simulink library "commsink2"  (Simulink 6.0)
settings: Solver=ode45  SolverMode=SingleTasking  StartTime=0.0  StopTime=10.0  RelTol=1e-3
undefined symbols (not defined in the file or in its folder): commblkeyescat2, get, sdspfscope2
libraries: simulink x6, dspsigattribs x6, dspbuff3 x3, dspsnks4 x3, dspsrcs4 x3, dspsigops x3
settings Model: CovMetricSettings=d  Creator=tdelve  LastModifiedBy=mmclerno  ExtModeAutoUpdateStatusClock=off  UpdateModelReferenceTargets=IfOutOfDate
settings Model: ForwardingTableString=|
  | ||__slOldName__||commsink2/Continuous-Time
  | Eye and Scatter
  | Diagrams||__slNewName__||cbobsv2p5/Continuous-Time
  | Eye and Scatter
  | Diagrams||__slOldName__||commsink2/Triggered Write to File||__slNewName__||cbobsv2p5/Triggered Write to File||__slOldName__||commsink2/Error Rate Calculation||__slNewName__||commsink2/Error Rate
  | Calculation||__slOldName__||commsink2/Discrete-Time
  | Eye and Scatter
  | Diagrams||__slNewName__||cbobsv2/Discrete-Time
  | Eye and Scatter
  | Diagrams
settings DataIOCC: SignalLoggingName=logsOut
settings OptimizationCC: BooleanDataType=off
settings DebuggingCC: CheckExecutionContextPreStartOutputMsg=on  CheckExecutionContextRuntimeOutputMsg=on  SolverPrmCheckMsg=none
settings HardwareCC: TargetUnknown=on
settings ModelReferenceCC: UpdateModelReferenceTargets=IfOutOfDate
settings GRTTargetCC: UtilityFuncGeneration=Automatic  LifeSpan=inf
settings SFSimCC: SFSimApplyToAllLibs=on  SFSimBuildMode=Incremental

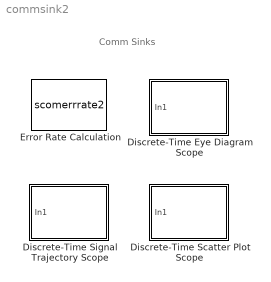
== system commsink2 ==
  note: Comm Sinks
  Discrete-Time Eye Diagram Scope : Subsystem  Tag=EyeDiagram  LoadFcn=commblkeyescat2(gcb,'Load');  StopFcn=sdspfscope2([],[],[],'StopBlock',[],[]);  EnableExecutionContextPropagation=on  mask(Discrete-Time Eye Diagram Scope){sampPerSymb=8, offsetEye=0, symbPerTrace=1, numTraces=40, numNewFrames=10, LineMarkers=, LineStyles=-, LineColors=b, dupPoints=on, fading=on, render=on, AxisGrid=on, yMin=-1.5, yMax=1.5, inphaseLabel=In-phase Amplitude, quadratureLabel=Quadrature Amplitude, openScopeAtSimStart=on, dispDiagram=In-phase and Quadrature, FrameNumber=off, FigPos=get(0,'defaultfigureposition');, figTitle=Eye Diagram, block_type_=eye, numLinesMax=8}
      mask prompts: sampPerSymb "Samples per symbol:"; offsetEye "Offset (samples):"; symbPerTrace "Symbols per trace:"; numTraces "Traces displayed:"; numNewFrames "New traces per display:"; LineMarkers "Markers:"; LineStyles "Line style:"; LineColors "Line color:"; dupPoints "Duplicate points at trace boundary"; fading "Color fading"; render "High quality rendering"; AxisGrid "Show grid"; yMin "Y axis minimum:"; yMax "Y axis maximum:"; inphaseLabel "In-phase Y-axis label:"; quadratureLabel "Quadrature Y-axis label:"; openScopeAtSimStart "Open scope at start of simulation"; dispDiagram "Eye diagram to display:"; FrameNumber "Trace number"; FigPos "Scope position:"; figTitle "Title:"; block_type_ "Block select"; numLinesMax "Max Num Lines"
      mask help:
      | The Discrete-Time Eye Diagram Scope displays multiple traces of a modulated signal to reveal the modulation characteristics such as pulse shaping, as well as channel distortions of the signal.
      |
      |
      | The signal is divided into traces with length, 'Samples per symbol'  * 'Symbols per trace' starting by skipping 'Offset' samples at the beginning.
      mask init:
      | commblkeyescat2(gcb,'init','eye');
      settings: OpenFcn=dspblkfscope2('dynamic','OpenScope');
      mask Help: helpview(commbhelp)
      mask StyleString: edit,edit,edit,edit,edit,edit,edit,edit,checkbox,checkbox,checkbox,checkbox,edit,edit,edit,edit,checkbox,popup(In-phase Only|In-phase and Quadrature),checkbox,edit,edit,popup(eye|scatter|xy),edit
      mask CallbackString: |||||||||||||||||commblkeyescat2(gcb,'cbDispDiagram');|||||
      mask TabNameString: Plotting Properties,Plotting Properties,Plotting Properties,Plotting Properties,Plotting Properties,Rendering Properties,Rendering Properties,Rendering Properties,Rendering Properties,Rendering Properties,Rendering Properties,Rendering Properties,Axes Properties,Axes Properties,Axes Properties,Axes Properties,Figure Properties,Figure Properties,Figure Properties,Figure Properties,Figure Properties,Figure Properties,Figure Properties
      mask Display: image(imread('eye.bmp','bmp'),'center')
  Discrete-Time Scatter Plot Scope : Subsystem  Tag=ScatterPlot  LoadFcn=commblkeyescat2(gcb,'Load');  StopFcn=sdspfscope2([],[],[],'StopBlock',[],[]);  EnableExecutionContextPropagation=on  mask(Discrete-Time Scatter Plot Scope){sampPerSymb=1, offsetEye=0, numTraces=40, numNewFrames=10, LineMarkers=., LineStyles=, LineColors=b, fading=on, render=on, AxisGrid=on, xMin=-1.5, xMax=1.5, yMin=-1.5, yMax=1.5, inphaseLabel=In-phase Amplitude, quadratureLabel=Quadrature Amplitude, openScopeAtSimStart=on, FrameNumber=off, FigPos=get(0,'defaultfigureposition');, figTitle=Scatter Plot, numLinesMax=8, block_type_=scatter}
      mask prompts: sampPerSymb "Samples per symbol:"; offsetEye "Offset (samples):"; numTraces "Points displayed:"; numNewFrames "New points per display:"; LineMarkers "Markers:"; LineStyles "Line style:"; LineColors "Line color:"; fading "Color fading"; render "High quality rendering"; AxisGrid "Show grid"; xMin "X-axis minimum:"; xMax "X-axis maximum:"; yMin "Y-axis minimum:"; yMax "Y axis maximum:"; inphaseLabel "In-phase X-axis label:"; quadratureLabel "Quadrature Y-axis label:"; openScopeAtSimStart "Open scope at start of simulation"; FrameNumber "Point number"; FigPos "Scope position:"; figTitle "Title:"; numLinesMax "Max Num Lines"; block_type_ "Block Type"
      mask help:
      | The Discrete-Time Scatter Plot Scope is used to display a modulated signal constellation in its signal space by plotting the In-phase component versus the Quadrature component.
      |
      |
      | Use with 'Samples per Symbol' set to 1 to view signals after detection or for signals without oversampling.  For oversampled signals, the input is decimated by 'Samples per symbol' skipping 'Offset' initial samples.
      mask init:
      | x = [2 8 5 2 8 5 5 5];
      | y = [2 8 5 8 2 5 8 2];
      | commblkeyescat2(gcb,'init','scatter');
      settings: OpenFcn=dspblkfscope2('dynamic','OpenScope');
      mask Help: helpview(commbhelp)
      mask StyleString: edit,edit,edit,edit,edit,edit,edit,checkbox,checkbox,checkbox,edit,edit,edit,edit,edit,edit,checkbox,checkbox,edit,edit,edit,popup(eye|scatter|xy)
      mask TabNameString: Plotting Properties,Plotting Properties,Plotting Properties,Plotting Properties,Rendering Properties,Rendering Properties,Rendering Properties,Rendering Properties,Rendering Properties,Rendering Properties,Axes Properties,Axes Properties,Axes Properties,Axes Properties,Axes Properties,Axes Properties,Figure Properties,Figure Properties,Figure Properties,Figure Properties,Figure Properties,Figure Properties
      mask Display: image(imread('scatter.bmp','bmp'),'center')
  Discrete-Time Signal Trajectory Scope : Subsystem  Tag=SignalTrajectory  LoadFcn=commblkeyescat2(gcb,'Load');  StopFcn=sdspfscope2([],[],[],'StopBlock',[],[]);  EnableExecutionContextPropagation=on  mask(Discrete-Time Signal Trajectory Scope){sampPerSymb=8, offsetEye=0, numTraces=40, numNewFrames=10, LineMarkers=, LineStyles=-, LineColors=b, fading=on, render=on, AxisGrid=on, xMin=-1.5, xMax=1.5, yMin=-1.5, yMax=1.5, inphaseLabel=In-phase Amplitude, quadratureLabel=Quadrature Amplitude, openScopeAtSimStart=on, FrameNumber=off, FigPos=get(0,'defaultfigureposition');, figTitle=Signal Trajectory, numLinesMax=8, block_type_=xy}
      mask prompts: sampPerSymb "Samples per symbol:"; offsetEye "Offset (samples):"; numTraces "Symbols displayed:"; numNewFrames "New symbols per display:"; LineMarkers "Markers:"; LineStyles "Line style:"; LineColors "Line color:"; fading "Color fading"; render "High quality rendering"; AxisGrid "Show grid"; xMin "X-axis minimum:"; xMax "X-axis maximum:"; yMin "Y-axis minimum:"; yMax "Y axis maximum:"; inphaseLabel "In-phase X-axis label:"; quadratureLabel "Quadrature Y-axis label:"; openScopeAtSimStart "Open scope at start of simulation"; FrameNumber "Symbol number"; FigPos "Scope position:"; figTitle "Title:"; numLinesMax "Max Num Lines"; block_type_ "Block Type"
      mask help: The Discrete-Time Signal Trajectory Scope is used to display a modulated signal constellation in its signal space by plotting the In-phase component versus the Quadrature component.
      mask init:
      | x = [2 8 5 2 8 5 5 5];
      | y = [2 8 5 8 2 5 8 2];
      | commblkeyescat2(gcb,'init','xy');
      settings: OpenFcn=dspblkfscope2('dynamic','OpenScope');
      mask Help: helpview(commbhelp)
      mask StyleString: edit,edit,edit,edit,edit,edit,edit,checkbox,checkbox,checkbox,edit,edit,edit,edit,edit,edit,checkbox,checkbox,edit,edit,edit,popup(eye|scatter|xy)
      mask TabNameString: Plotting Properties,Plotting Properties,Plotting Properties,Plotting Properties,Rendering Properties,Rendering Properties,Rendering Properties,Rendering Properties,Rendering Properties,Rendering Properties,Axes Properties,Axes Properties,Axes Properties,Axes Properties,Axes Properties,Axes Properties,Figure Properties,Figure Properties,Figure Properties,Figure Properties,Figure Properties,Figure Properties
      mask Display: image(imread('sig_traj.bmp','bmp'),'center')
  Error Rate Calculation : S-Function  FunctionName=scomerrrate2  Parameters=N, st_delay, cp_mode, subframe, PMode, WsName, RsMode2,stop,numErr,maxBits  mask(Error Rate Calculation){N=0, st_delay=0, cp_mode=Entire frame, subframe=[], PMode=Workspace, WsName=ErrorVec, RsMode2=off, stop=off, numErr=100, maxBits=1e6}
      mask prompts: N "Receive delay:"; st_delay "Computation delay:"; cp_mode "Computation mode:"; subframe "Selected samples from frame:"; PMode "Output data:"; WsName "Variable name:"; RsMode2 "Reset port"; stop "Stop simulation"; numErr "Target number of errors:"; maxBits "Maximum number of symbols:"
      mask help:
      | Compute the error rate of the received data by comparing it to a delayed version of the transmitted data. The block output is a three-element vector consisting of the error rate, followed by the number of errors detected and the total number of symbols compared. This vector can be sent to either the workspace or an output port.
      |
      | The delays are specified in number of samples, regardless of whether the input is a scalar or a vector. The inputs to the 'Tx' and 'Rx' ports must be sample-based scalars or frame-based column vectors.
      |
      | The 'Stop simulation' option stops the simulation upon detecting a target number of errors or a maximum number of symbols, whichever comes first.
      mask init:
      | [s] = commblkerrrate(gcb,'init');
      | if(PMode==1)
      |     if(isempty(WsName))
      |         error('Output variable name cannot be empty.')
      |     end
      |     if(~isletter(WsName(1)))
      |         error('Output variable name must be a string.')
      |     end
      | end
      mask Help: helpview(commbhelp)
      mask StyleString: edit,edit,popup(Entire frame|Select samples from mask|Select samples from port),edit,popup(Workspace|Port),edit,checkbox,checkbox,edit,edit
      mask CallbackString: ||commblkerrrate(gcb,'CpMode');||commblkerrrate(gcb,'OutMode');|||commblkerrrate(gcb,'UpdateEnables');||
      mask Display:
      | disp('  Error Rate\n  Calculation');
      | port_label('input',s.i1,s.i1s);
      | port_label('input',s.i2,s.i2s);
      | port_label('input',s.i3,s.i3s);
      | port_label('input',s.i4,s.i4s);

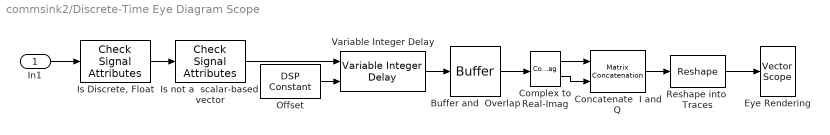
== system commsink2/Discrete-Time Eye Diagram Scope ==
  In1 : Inport  LatchInput=off
  Buffer and  Overlap : dspbuff3/Buffer  N=numTraces * sampPerSymb * symbPerTrace  V=(numTraces - numNewFrames)* sampPerSymb  ic=0
  Complex to Real-Imag : ComplexToRealImag
  Concatenate  I and Q : simulink/Math Operations/Matrix Concatenation  numInports=2  catMethod=Horizontal
  Eye Rendering : dspsnks4/Vector Scope  ScopeProperties=on  Domain=Time  HorizSpan=1  DisplayProperties=off  AxisGrid=on  Memory=off  FrameNumber=on  AxisLegend=off  AxisZoom=off  OpenScopeAtSimStart=on  OpenScopeImmediately=off  FigPos=FigPos  AxisProperties=off  XUnits=Hertz  XRange=[0...Fs/2]  InheritXIncr=on  XIncr=1  XLabel=Time  YUnits=dB  YLabel=Amplitude  LineProperties=off
      settings: YMin=-1.5  YMax=1.5
  "Is Discrete, Float" : dspsigattribs/Check Signal Attributes  SigAttribCheckMethod=Does not match attributes exactly  Complexity=Ignore  Frame=Ignore  DimsCheckMethod=Is...  Dimensions=Vector (1-D or 2-D) or scalar  DatatypeCheckMethod=Is...  DatatypeGeneral=Floating-point  DtypeFloatSpecific=Any floating-point  DtypeFixedSpecific=Any fixed-point  DtypeIntSpecific=Any integer  SampleMode=Discrete
  Is not a  scalar-based  vector : dspsigattribs/Check Signal Attributes  SigAttribCheckMethod=Matches attributes exactly  Complexity=Ignore  Frame=Sample-based  DimsCheckMethod=Is...  Dimensions=Vector (1-D or 2-D)  DatatypeCheckMethod=Ignore  DatatypeGeneral=Floating-point  DtypeFloatSpecific=Any floating-point  DtypeFixedSpecific=Any fixed-point  DtypeIntSpecific=Any integer  SampleMode=Ignore
  Offset : dspsrcs4/DSP Constant  Value=offsetEye + round(sampPerSymb/2)  SampleMode=Discrete  discreteOutput=Sample-based  continuousOutput=Sample-based  sampTime=-1  framePeriod=-1  dataType=Inherit from 'Constant value'  isSigned=on  wordLen=16  udDataType=sfix(16)  fracBitsMode=Best precision  numFracBits=15  InterpretAs1D=off  Ts=-1  FramebasedOutput=off
  Reshape into  Traces : simulink/Math Operations/Reshape  OutputDimensionality=Customize  OutputDimensions=[sampPerSymb*symbPerTrace, (numTraces*2)]
  Variable Integer Delay : dspsigops/Variable Integer Delay  dmax=100  ic=0
  wires:
  Is not a  scalar-based  vector/1 -> Variable Integer Delay/1
  "Is Discrete, Float"/1 -> Is not a  scalar-based  vector/1
  Reshape into  Traces/1 -> Eye Rendering/1
  Complex to Real-Imag/2 -> Concatenate  I and Q/2
  Complex to Real-Imag/1 -> Concatenate  I and Q/1
  Concatenate  I and Q/1 -> Reshape into  Traces/1
  Buffer and  Overlap/1 -> Complex to Real-Imag/1
  Offset/1 -> Variable Integer Delay/2
  In1/1 -> "Is Discrete, Float"/1
  Variable Integer Delay/1 -> Buffer and  Overlap/1

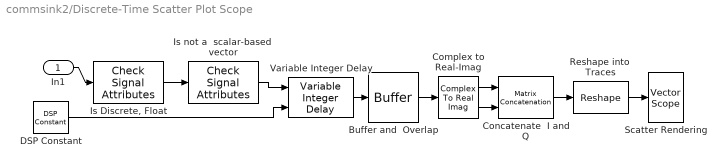
== system commsink2/Discrete-Time Scatter Plot Scope ==
  In1 : Inport  LatchInput=off
  Buffer and  Overlap : dspbuff3/Buffer  N=numTraces * sampPerSymb  V=(numTraces - numNewFrames)* sampPerSymb  ic=0
  Complex to Real-Imag : ComplexToRealImag
  Concatenate  I and Q : simulink/Math Operations/Matrix Concatenation  numInports=2  catMethod=Horizontal
  DSP Constant : dspsrcs4/DSP Constant  Value=offsetEye+sampPerSymb-1  SampleMode=Discrete  discreteOutput=Sample-based  continuousOutput=Sample-based  sampTime=-1  framePeriod=-1  dataType=Inherit from 'Constant value'  isSigned=on  wordLen=16  udDataType=sfix(16)  fracBitsMode=Best precision  numFracBits=15  InterpretAs1D=off  Ts=-1  FramebasedOutput=off
  "Is Discrete, Float" : dspsigattribs/Check Signal Attributes  SigAttribCheckMethod=Does not match attributes exactly  Complexity=Complex  Frame=Ignore  DimsCheckMethod=Is...  Dimensions=Vector (1-D or 2-D) or scalar  DatatypeCheckMethod=Is...  DatatypeGeneral=Floating-point  DtypeFloatSpecific=Any floating-point  DtypeFixedSpecific=Any fixed-point  DtypeIntSpecific=Any integer  SampleMode=Discrete
  Is not a  scalar-based  vector : dspsigattribs/Check Signal Attributes  SigAttribCheckMethod=Matches attributes exactly  Complexity=Ignore  Frame=Sample-based  DimsCheckMethod=Is...  Dimensions=Vector (1-D or 2-D)  DatatypeCheckMethod=Ignore  DatatypeGeneral=Floating-point  DtypeFloatSpecific=Any floating-point  DtypeFixedSpecific=Any fixed-point  DtypeIntSpecific=Any integer  SampleMode=Ignore
  Reshape into  Traces : simulink/Math Operations/Reshape  OutputDimensionality=Customize  OutputDimensions=[sampPerSymb, (numTraces*2)]
  Scatter Rendering : dspsnks4/Vector Scope  ScopeProperties=on  Domain=User-defined  HorizSpan=1  DisplayProperties=off  AxisGrid=on  Memory=off  FrameNumber=on  AxisLegend=off  AxisZoom=off  OpenScopeAtSimStart=on  OpenScopeImmediately=off  FigPos=FigPos  AxisProperties=off  XUnits=Hertz  XRange=[0...Fs/2]  InheritXIncr=on  XIncr=1  XLabel=Time  YUnits=dB  YLabel=Quadrature Amplitude  LineProperties=off  LineDisables=on
      settings: YMin=-1.5  YMax=1.5
  Variable Integer Delay : dspsigops/Variable Integer Delay  dmax=100  ic=0
  wires:
  Complex to Real-Imag/1 -> Concatenate  I and Q/1
  Complex to Real-Imag/2 -> Concatenate  I and Q/2
  Concatenate  I and Q/1 -> Reshape into  Traces/1
  Reshape into  Traces/1 -> Scatter Rendering/1
  Buffer and  Overlap/1 -> Complex to Real-Imag/1
  Variable Integer Delay/1 -> Buffer and  Overlap/1
  DSP Constant/1 -> Variable Integer Delay/2
  "Is Discrete, Float"/1 -> Is not a  scalar-based  vector/1
  Is not a  scalar-based  vector/1 -> Variable Integer Delay/1
  In1/1 -> "Is Discrete, Float"/1

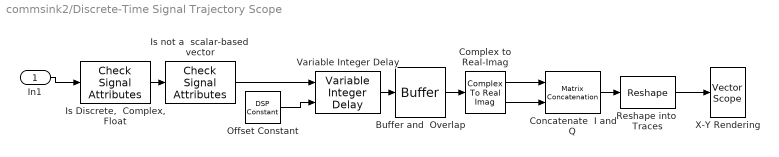
== system commsink2/Discrete-Time Signal Trajectory Scope ==
  In1 : Inport  LatchInput=off
  Buffer and  Overlap : dspbuff3/Buffer  N=numTraces * sampPerSymb  V=(numTraces - numNewFrames)* sampPerSymb  ic=0
  Complex to Real-Imag : ComplexToRealImag
  Concatenate  I and Q : simulink/Math Operations/Matrix Concatenation  numInports=2  catMethod=Horizontal
  "Is Discrete,  Complex, Float" : dspsigattribs/Check Signal Attributes  SigAttribCheckMethod=Does not match attributes exactly  Complexity=Complex  Frame=Ignore  DimsCheckMethod=Is...  Dimensions=Vector (1-D or 2-D) or scalar  DatatypeCheckMethod=Is...  DatatypeGeneral=Floating-point  DtypeFloatSpecific=Any floating-point  DtypeFixedSpecific=Any fixed-point  DtypeIntSpecific=Any integer  SampleMode=Discrete
  Is not a  scalar-based  vector : dspsigattribs/Check Signal Attributes  SigAttribCheckMethod=Matches attributes exactly  Complexity=Ignore  Frame=Sample-based  DimsCheckMethod=Is...  Dimensions=Vector (1-D or 2-D)  DatatypeCheckMethod=Ignore  DatatypeGeneral=Floating-point  DtypeFloatSpecific=Any floating-point  DtypeFixedSpecific=Any fixed-point  DtypeIntSpecific=Any integer  SampleMode=Ignore
  Offset Constant : dspsrcs4/DSP Constant  Value=offsetEye + round(sampPerSymb/2)  SampleMode=Discrete  discreteOutput=Sample-based  continuousOutput=Sample-based  sampTime=-1  framePeriod=-1  dataType=Inherit from 'Constant value'  isSigned=on  wordLen=16  udDataType=sfix(16)  fracBitsMode=Best precision  numFracBits=15  InterpretAs1D=off  Ts=-1  FramebasedOutput=off
  Reshape into  Traces : simulink/Math Operations/Reshape  OutputDimensionality=Customize  OutputDimensions=[sampPerSymb, (numTraces*2)]
  Variable Integer Delay : dspsigops/Variable Integer Delay  dmax=100  ic=0
  X-Y Rendering : dspsnks4/Vector Scope  ScopeProperties=on  Domain=User-defined  HorizSpan=1  DisplayProperties=off  AxisGrid=on  Memory=off  FrameNumber=on  AxisLegend=off  AxisZoom=off  OpenScopeAtSimStart=on  OpenScopeImmediately=off  FigPos=FigPos  AxisProperties=off  XUnits=Hertz  XRange=[0...Fs/2]  InheritXIncr=on  XIncr=1  XLabel=In-phase Amplitude  YUnits=dB  YLabel=Quadrature Amplitude  LineProperties=off  LineDisables=on
      settings: YMin=-1.5  YMax=1.5
  wires:
  In1/1 -> "Is Discrete,  Complex, Float"/1
  Is not a  scalar-based  vector/1 -> Variable Integer Delay/1
  "Is Discrete,  Complex, Float"/1 -> Is not a  scalar-based  vector/1
  Offset Constant/1 -> Variable Integer Delay/2
  Variable Integer Delay/1 -> Buffer and  Overlap/1
  Buffer and  Overlap/1 -> Complex to Real-Imag/1
  Reshape into  Traces/1 -> X-Y Rendering/1
  Concatenate  I and Q/1 -> Reshape into  Traces/1
  Complex to Real-Imag/2 -> Concatenate  I and Q/2
  Complex to Real-Imag/1 -> Concatenate  I and Q/1
